simulink model "q2"  (R2020a)
settings: Solver=VariableStepAuto  StartTime=0.0  StopTime=10.0  RelTol=1e-3
values from neighbouring files (symbols this model uses):
  B = 500    [dummy_signal.m]
  K1 = 5000    [dummy_signal.m]
  K2 = 250000    [dummy_signal.m]
  M1 = 2000    [dummy_signal.m]
  M2 = 500    [dummy_signal.m]
settings Model: Creator=kiran  LastModifiedBy=kiran
settings DataIOCC: ExternalInput=[t, stin]  LoadExternalInput=on

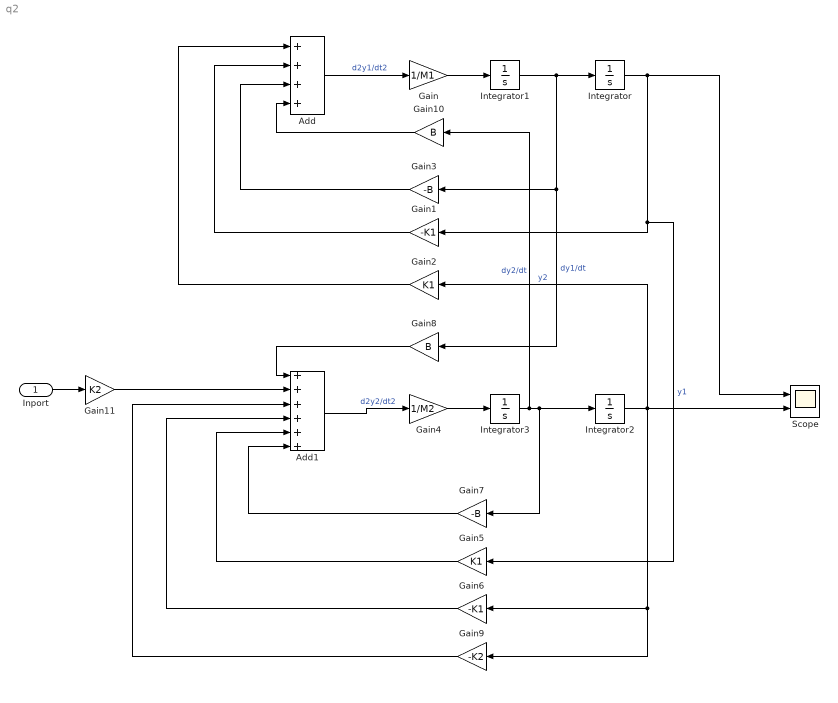
== system q2 ==
  Inport : Inport
  Add : Sum  Inputs=++++
  Add1 : Sum  Inputs=++++++
  Gain : Gain  Gain=1/M1
  Gain1 : Gain  Gain=-K1
  Gain10 : Gain  Gain=B
  Gain11 : Gain  Gain=K2
  Gain2 : Gain  Gain=K1
  Gain3 : Gain  Gain=-B
  Gain4 : Gain  Gain=1/M2
  Gain5 : Gain  Gain=K1
  Gain6 : Gain  Gain=-K1
  Gain7 : Gain  Gain=-B
  Gain8 : Gain  Gain=B
  Gain9 : Gain  Gain=-K2
  Integrator{,1..3} (4 alike) : Integrator
  Scope : Scope  NumInputPorts=2
  wires:
  Add/1 -> Gain/1  "d2y1/dt2"
  Gain/1 -> Integrator1/1
  Integrator1/1 -> Integrator/1, Gain3/1, Gain8/1  "dy1/dt"
  Integrator/1 -> Gain1/1, Gain5/1, Scope/1  "y1"
  Gain2/1 -> Add/1
  Gain1/1 -> Add/2
  Gain3/1 -> Add/3
  Integrator2/1 -> Scope/2, Gain2/1, Gain9/1, Gain6/1  "y2"
  Gain4/1 -> Integrator3/1
  Integrator3/1 -> Gain7/1, Integrator2/1, Gain10/1  "dy2/dt"
  Add1/1 -> Gain4/1  "d2y2/dt2"
  Gain10/1 -> Add/4
  Inport/1 -> Gain11/1
  Gain8/1 -> Add1/1
  Gain11/1 -> Add1/2
  Gain9/1 -> Add1/3
  Gain6/1 -> Add1/4
  Gain7/1 -> Add1/6
  Gain5/1 -> Add1/5
